simulink model "pezg"  (R2012b)
settings: Solver=ode45  StartTime=0.0  StopTime=30  RelTol=1e-3
undefined symbols (not defined in the file): pez
settings Model: Creator=Daniel  LastModifiedBy=Daniel

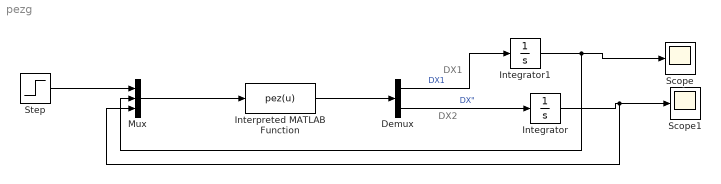
== system pezg ==
  note: DX2
  note: DX1
  Demux : Demux  Outputs=2
  Integrator : Integrator
  Integrator1 : Integrator  InitialCondition=pi/2
  Interpreted MATLAB Function : MATLABFcn  MATLABFcn=pez(u)  OutputDimensions=2
  Mux : Mux  Inputs=3
  Scope : Scope
  Scope1 : Scope
  Step : Step  After=10  SampleTime=0
  wires:
  Interpreted MATLAB Function/1 -> Demux/1
  Mux/1 -> Interpreted MATLAB Function/1
  Demux/1 -> Integrator1/1  "DX1"
  Demux/2 -> Integrator/1  "DX\""
  Step/1 -> Mux/1
  Integrator1/1 -> Mux/2, Scope/1
  Integrator/1 -> Mux/3, Scope1/1
